simulink model "TADPOLE_Open_Loop"  (R2024b)
settings: Solver=VariableStepAuto  StartTime=0.0  StopTime=20  RelTol=1e-3
settings Model: Creator=pplat  LastModifiedBy=rober
settings DebuggingCC: AlgebraicLoopMsg=none

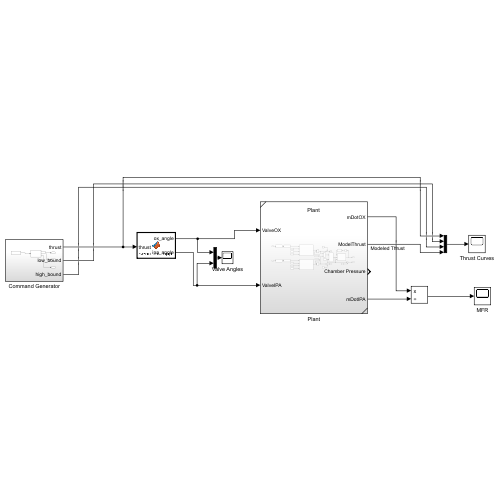
[thumbnail: Simulink's stored preview of the top-level diagram]
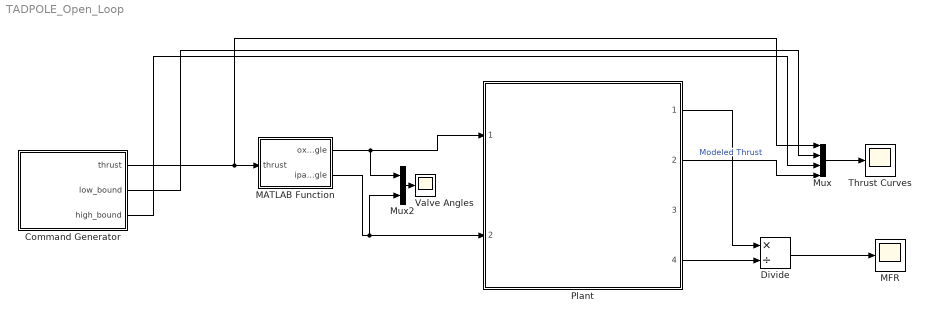
== system TADPOLE_Open_Loop ==
  Command Generator : Subsystem
  Divide : Product  Inputs=*/
  MATLAB Function : MATLAB Function  TreatAsAtomicUnit=on
  MFR : Scope
  Mux : Mux
  Mux2 : Mux  Inputs=2
  Plant : Subsystem  ReferencedSubsystem=Plant
  Thrust Curves : Scope
  Valve Angles : Scope
  wires:
  Mux/1 -> Thrust Curves/1
  Plant/1 -> Divide/1
  Plant/4 -> Divide/2
  MATLAB Function/2(ipa_angle) -> Plant/2, Mux2/2
  MATLAB Function/1(ox_angle) -> Plant/1, Mux2/1
  Mux2/1 -> Valve Angles/1
  Divide/1 -> MFR/1
  Command Generator/1(thrust) -> Mux/1, MATLAB Function/1(thrust)
  Plant/2 -> Mux/4  "Modeled Thrust"
  Command Generator/2(low_bound) -> Mux/2
  Command Generator/3(high_bound) -> Mux/3

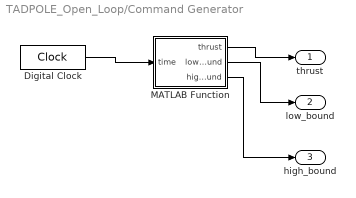
== system TADPOLE_Open_Loop/Command Generator ==
  Digital Clock : DigitalClock  SampleTime=1/60
  MATLAB Function : MATLAB Function  TreatAsAtomicUnit=on
  thrust : Outport
  low_bound : Outport  Port=2
  high_bound : Outport  Port=3
  wires:
  MATLAB Function/1(thrust) -> thrust/1
  Digital Clock/1 -> MATLAB Function/1(time)
  MATLAB Function/2(low_bound) -> low_bound/1
  MATLAB Function/3(high_bound) -> high_bound/1

== matlab function TADPOLE_Open_Loop/Command Generator/MATLAB Function ==
  data: time input; thrust output; low_bound output; high_bound output
function [thrust,low_bound,high_bound] = thrustCurveBounds(time)
thrust = thrustCurve(time);
t_past = thrustCurve(time - 0.5);
t_future = thrustCurve(time + 0.5);

high_bound = max([thrust, t_past, t_future]) + 0.05 * 550;
low_bound = min([thrust, t_past, t_future]) - 0.05 * 550;

end

== matlab function TADPOLE_Open_Loop/MATLAB Function ==
  data: thrust input; ox_angle output; ipa_angle output
function [ox_angle, ipa_angle] = send_to_cpp(thrust)
coder.extrinsic('open_loop_valve_control_wrap');  % Declare MEX function as extrinsic
ox_angle = 0;
ipa_angle = 0;
[ox_angle, ipa_angle] = open_loop_valve_control_wrap(thrust);
